simulink model "ModelConveyor"  (R2020b)
settings: Solver=FixedStepAuto  StartTime=0.0  StopTime=10.0  FixedStep=0.010  RelTol=1e-3
settings Model: Creator=kaebi  LastModifiedBy=kaebi
settings OptimizationCC: DefaultParameterBehavior=Inlined  LocalBlockOutputs=off
settings RTWCC: Description=TwinCAT GRT Target  SystemTargetFile=TwinCatGrt.tlc  TemplateMakefile=tcgrt_msbuild.tmf  TargetLang=C++
settings STFCustomTargetCC: TargetLangStandard=C++03 (ISO)  ConcurrentExecutionCompliant=off  CombineOutputUpdateFcns=on  CodeInterfacePackaging=Reusable function  GRTInterface=off  GenerateAllocFcn=on  SystemTargetFile=TwinCatGrt.tlc
settings GRTTargetCC: TargetLangStandard=C++03 (ISO)  ParMdlRefBuildCompliant=off  CompOptLevelCompliant=off  ConcurrentExecutionCompliant=off  MatFileLogging=off  CodeInterfacePackaging=Reusable function  GenerateAllocFcn=on  UseToolchainInfoCompliant=off  ExtModeMexFile=TcExtModeClient
settings ConfigComp: PLC_TargetIDE=codesys23

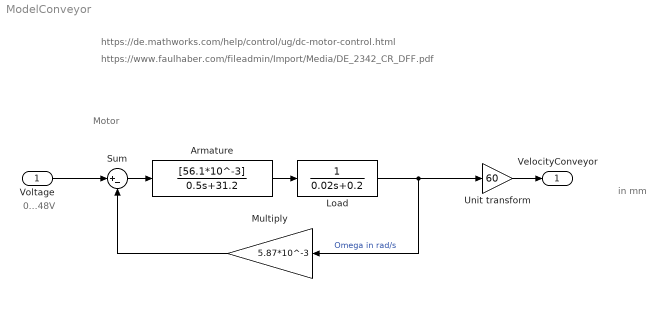
== system ModelConveyor ==
  note: in mm
  note: 0...48V
  note: Motor
  note: https://www.faulhaber.com/fileadmin/Import/Media/DE_2342_CR_DFF.pdf
  note: https://de.mathworks.com/help/control/ug/dc-motor-control.html
  Voltage : Inport
  Armature : TransferFcn  Numerator=[56.1*10^-3]  Denominator=[0.5 31.2]
  Load : TransferFcn  Denominator=[0.02 0.2]
  Multiply : Gain  Gain=5.87*10^-3
  Sum : Sum  Inputs=|+-
  Unit transform : Gain  Gain=60
  VelocityConveyor : Outport
  wires:
  Voltage/1 -> Sum/1
  Armature/1 -> Load/1
  Sum/1 -> Armature/1
  Load/1 -> Unit transform/1, Multiply/1  "Omega in rad/s"
  Multiply/1 -> Sum/2
  Unit transform/1 -> VelocityConveyor/1
